simulink model "PID_Controller_ROS2023a"  (R2023a)
settings: Solver=VariableStepAuto  StartTime=0.0  StopTime=60  RelTol=1e-3
libraries: robotlib x3, slpidlib x1
settings Model: Creator=abbas  LastModifiedBy=abbas

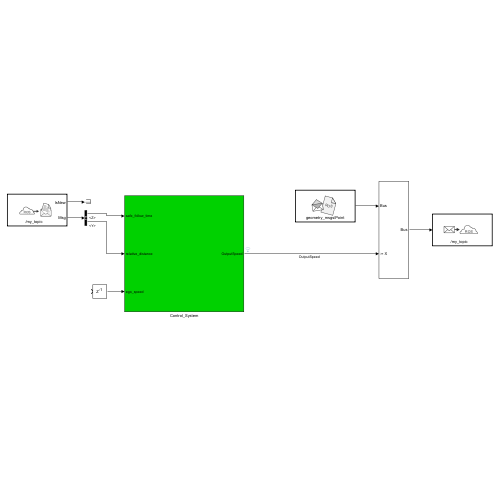
[thumbnail: Simulink's stored preview of the top-level diagram]
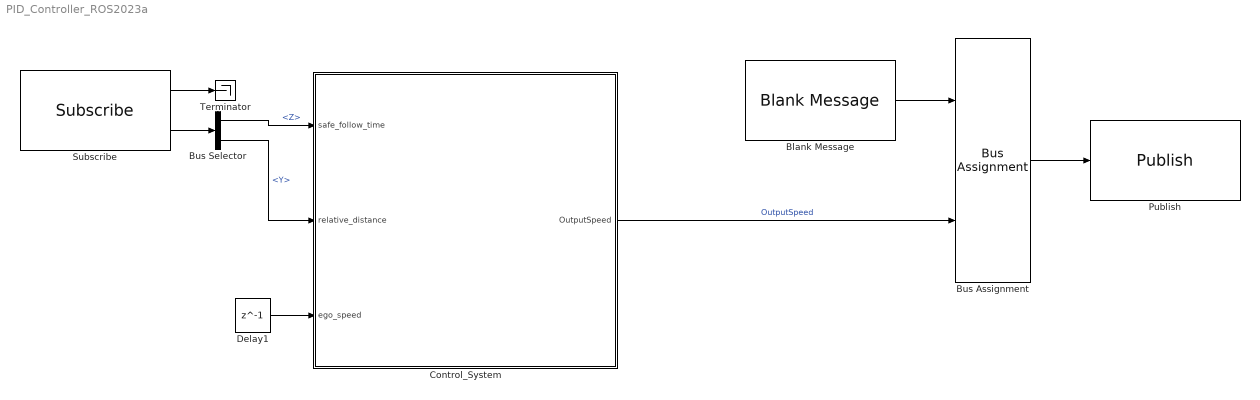
== system PID_Controller_ROS2023a ==
  Blank Message : robotlib/Blank Message  messageClass=Message  entityType=geometry_msgs/Point  messageType=geometry_msgs/Point  SampleTime=inf  legacyBusStruct=off
  Bus Assignment : BusAssignment  AssignedSignals=X
  Bus Selector : BusSelector  OutputSignals=Z,Y
  Control_System : Subsystem
  Delay1 : Delay  DelayLength=1  InitialCondition=0
  Publish : robotlib/Publish  topicSource=Select from ROS network  topic=/my_topic  messageType=geometry_msgs/Point  legacyBusStruct=off  messageQueueLength=1
  Subscribe : robotlib/Subscribe  topicSource=Specify your own  topic=/my_topic  messageType=geometry_msgs/Point  SampleTime=-1  legacyBusStruct=off  messageQueueLength=1
  Terminator : Terminator
  wires:
  Control_System/1(OutputSpeed) -> Bus Assignment/2  "OutputSpeed"
  Delay1/1 -> Control_System/3(ego_speed)
  Subscribe/2 -> Bus Selector/1
  Blank Message/1 -> Bus Assignment/1
  Bus Assignment/1 -> Publish/1
  Bus Selector/2 -> Control_System/2(relative_distance)  "<Y>"
  Bus Selector/1 -> Control_System/1(safe_follow_time)  "<Z>"
  Subscribe/1 -> Terminator/1

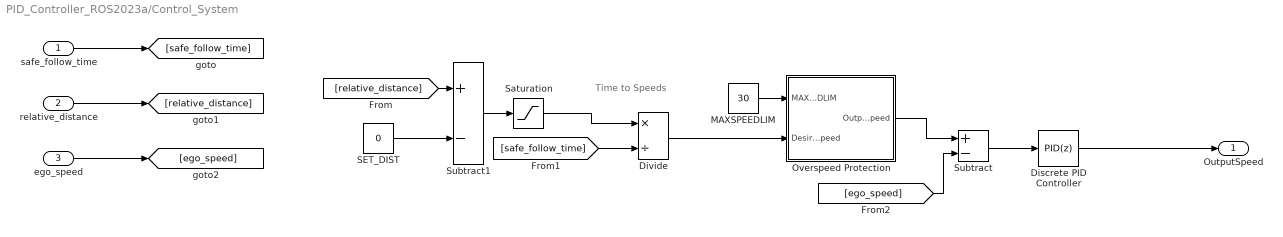
== system PID_Controller_ROS2023a/Control_System ==
  note: Time to Speeds
  safe_follow_time : Inport
  relative_distance : Inport  Port=2
  ego_speed : Inport  Port=3
  Discrete PID Controller : slpidlib/PID Controller  Controller=PID  Form=Parallel  TimeDomain=Discrete-time  UseExternalTs=off  SampleTime=0.1  IntegratorMethod=Forward Euler  FilterMethod=Forward Euler  ControllerParametersSource=internal  P=1.2  I=1  UseKiTs=on  D=0  N=100  UseFilter=on  TunerSelectOption=Frequency Response Based  InitialConditionSource=internal  InitialConditionForIntegrator=0  InitialConditionForFilter=0  DifferentiatorICPrevScaledInput=0  ExternalReset=none  TrackingMode=off  Kt=1  LimitOutput=off  SatLimitsSource=internal  UpperSaturationLimit=inf  LowerSaturationLimit=-inf  LinearizeAsGain=off  AntiWindupMode=none  Kb=1  LimitIntegrator=off  UpperIntegratorSaturationLimit=inf  LowerIntegratorSaturationLimit=-inf  POutMin=[]  POutMax=[]  IOutMin=[]  IOutMax=[]  DOutMin=[]  DOutMax=[]  NOutMin=[]  NOutMax=[]  SumOutMin=[]  SumOutMax=[]  SaturationOutMin=[]  SaturationOutMax=[]  PParamMin=[]  PParamMax=[]  IParamMin=[]  IParamMax=[]  DParamMin=[]  DParamMax=[]  NParamMin=[]  NParamMax=[]  KbParamMin=[]  KbParamMax=[]  KtParamMin=[]  KtParamMax=[]  KbOutMin=[]  KbOutMax=[]  KtOutMin=[]  KtOutMax=[]  IntegratorOutMin=[]  IntegratorOutMax=[]  FilterOutMin=[]  FilterOutMax=[]  SumI1OutMin=[]  SumI1OutMax=[]  SumI2OutMin=[]  SumI2OutMax=[]  SumI3OutMin=[]  SumI3OutMax=[]  SumI4OutMin=[]  SumI4OutMax=[]  SumDOutMin=[]  SumDOutMax=[]  DifferentiatorOutMin=[]  DifferentiatorOutMax=[]  FilterDiffOutCoefMin=[]  FilterDiffOutCoefMax=[]  ReciprocalOutMin=[]  ReciprocalOutMax=[]  SumDenOutMin=[]  SumDenOutMax=[]  SumNumOutMin=[]  SumNumOutMax=[]  DivideOutMin=[]  DivideOutMax=[]  UdiffTsProdOutMin=[]  UdiffTsProdOutMax=[]  NTsProdOutMin=[]  NTsProdOutMax=[]  UintegralTsProdOutMin=[]  UintegralTsProdOutMax=[]  UngainTsProdOutMin=[]  UngainTsProdOutMax=[]  ClampingZeroOutDataTypeStr=Inherit: Inherit via back propagation  ClampingZeroOutMin=[]  ClampingZeroOutMax=[]  FilterDenConstantOutDataTypeStr=Inherit: Inherit via back propagation  FilterDenConstantOutMin=[]  FilterDenConstantOutMax=[]  PCopyOutDataTypeStr=Inherit: Inherit via back propagation  PCopyOutMin=[]  PCopyOutMax=[]  NCopyOutDataTypeStr=Inherit: Inherit via back propagation  NCopyOutMin=[]  NCopyOutMax=[]  IntegratorContinuousStateAttributes=''  IntegratorStateMustResolveToSignalObject=off  IntegratorRTWStateStorageClass=Auto  FilterContinuousStateAttributes=''  FilterStateMustResolveToSignalObject=off  FilterRTWStateStorageClass=Auto  ParallelPVariant=InternalParameters  IdealPVariant=Disabled  IVariant=InternalParameters  DVariant=InternalParameters  IntegratorVariant=Discrete  SatVariant=Disabled  AWVariant=Passthrough  PCopyVariant=Disabled  TRVariant=Disabled  FdbkBlocksVariant=Forward  IdealPFdbkVariant=Disabled  SatFdbkVariant=Disabled  DerivativeFilterVariant=ForwardEulerFilter  NVariant=InternalParameters  NCopyVariant=Disabled  FilterICVariant=InternalICsFilter  IntegratorICVariant=InternalICs  ExternalResetVariant=Disabled  TRSumVariant=Passthrough  SumFdbkVariant=Disabled  SumVariant=Sum_PID  TsampFilterVariant=InternalTs  TsampNgainVariant=Passthrough  TsampIntegralVariant=Disabled_SignalSpec  ExternalSaturationOutDataTypeStr=Inherit: Same as second input
      settings: LibrarySourceBlock=simulink/Discrete/Discrete PID Controller
  Divide : Product  Inputs=*/
  MAXSPEEDLIM : Constant  Value=30
  Overspeed Protection : MATLAB Function  TreatAsAtomicUnit=on
  SET_DIST : Constant  Value=0
  Saturation : Saturate  UpperLimit=inf  LowerLimit=0
  Subtract : Sum  Inputs=+-
  Subtract1 : Sum  Inputs=+-
  OutputSpeed : Outport
  wires:
  Subtract/1 -> Discrete PID Controller/1
  SET_DIST/1 -> Subtract1/2
  Subtract1/1 -> Saturation/1
  safe_follow_time/1 -> [safe_follow_time]
  [safe_follow_time] -> Divide/2
  relative_distance/1 -> [relative_distance]
  [relative_distance] -> Subtract1/1
  ego_speed/1 -> [ego_speed]
  [ego_speed] -> Subtract/2
  Saturation/1 -> Divide/1
  Divide/1 -> Overspeed Protection/2(DesiredSpeed)
  MAXSPEEDLIM/1 -> Overspeed Protection/1(MAXSPEEDLIM)
  Overspeed Protection/1(Output_Speed) -> Subtract/1
  Discrete PID Controller/1 -> OutputSpeed/1

== matlab function PID_Controller_ROS2023a/Control_System/Overspeed Protection ==
  data: MAXSPEEDLIM input; Output_Speed output; DesiredSpeed input
function Output_Speed  = fcn(MAXSPEEDLIM, DesiredSpeed)

if DesiredSpeed >= MAXSPEEDLIM
    Output_Speed = MAXSPEEDLIM;
elseif DesiredSpeed < 0
    Output_Speed = 0;
else 
    Output_Speed = DesiredSpeed;

end
